simulink library "Susp_AxleTA2PRNoSteer"  (R2023b)
settings: Solver=ode23t  StartTime=0.0  StopTime=10.0  RelTol=1e-3
undefined symbols (not defined in the file): Axle1D, AxleIn, Init, RaceFix, RaceSpin, Susp, Visual, X, Y, Z
libraries: sm_lib x46, Suspension_Utilities x10, Susp_Components x5, Linkage_Shock x2, Susp_AxleTA4Watts x2, Linkage_Spring x2, Linkage_Bumpstop x1, Susp_TwistBeam x1
(part 1 of 2)
Description:
  | Component of Simscape Vehicle Templates Library
  | 
  | Copyright 2018-2025 The MathWorks, Inc.
settings Model: Creator=mwalker  LastModifiedBy=smiller
settings SolverCC: AlgebraicLoopSolver=TrustRegion
settings DataIOCC: ReturnWorkspaceOutputs=off
settings DebuggingCC: UnconnectedInputMsg=warning  UnconnectedOutputMsg=warning  UnconnectedLineMsg=warning  ArithmeticOperatorsInVariantConditions=warning
settings ModelReferenceCC: EnableRefExpFcnMdlSchedulingChecks=on
settings SFSimCC: CustomCodeUndefinedFunction=UseInterfaceOnly

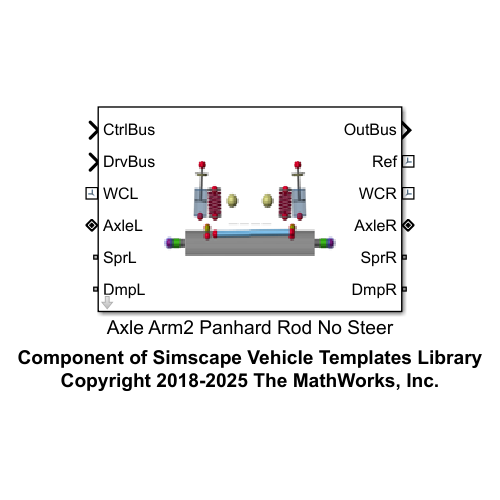
[thumbnail: Simulink's stored preview of the top-level diagram]
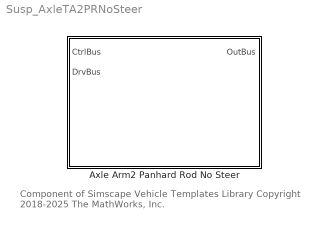
== system Susp_AxleTA2PRNoSteer ==
  note: Component of Simscape Vehicle Templates Library
      | Copyright 2018-2025 The MathWorks, Inc.
  Axle Arm2 Panhard Rod No Steer : Subsystem  VariantControl=LiveAxle  mask(Rigid Axle 2 Trailing Arm Panhard Rod Suspension, No Steer){Init=Init, hp_damper_topL=Susp.AxleTA2PR.Damper.sTopL.Value, hp_damper_topR=Susp.AxleTA2PR.Damper.sTopR.Value, hp_damper_botL=Susp.AxleTA2PR.Damper.sBottomL.Value, hp_damper_botR=Susp.AxleTA2PR.Damper.sBottomR.Value, hp_spring_topL=Susp.AxleTA2PR.Spring.sTopL.Value, hp_spring_topR=Susp.AxleTA2PR.Spring.sTopR.Value, hp_spring_botL=Susp.AxleTA2PR.Spring.sBottomL.Value, hp_spring_botR=Susp.AxleTA2PR.Spring.sBottomR.Value, hp_arm_body=Susp.AxleTA2PR.TrailingArm.sBody.Value, hp_arm_axleL=Susp.AxleTA2PR.TrailingArm.sAxleL.Value, hp_arm_axleR=Susp.AxleTA2PR.TrailingArm.sAxleR.Value, hp_pan_body=Susp.AxleTA2PR.PanhardRod.sBody.Value, hp_pan_axle=Susp.AxleTA2PR.PanhardRod.sAxle.Value, hp_axle_cg=Susp.AxleTA2PR.Axle.sCG.Value, hp_whl_ctrL=Susp.AxleTA2PR.Axle.sWheelCentreL.Value, hp_whl_ctrR=Susp.AxleTA2PR.Axle.sWheelCentreR.Value, hp_axle_outboardL=Susp.AxleTA2PR.Axle.sOutboardL.Value, hp_axle_outboardR=Susp.AxleTA2PR.Axle.sOutboardR.Value, hp_bumpstop_body=Susp.AxleTA2PR.Bumpstop.sBody.Value, hp_bumpstop_axle=Susp.AxleTA2PR.Bumpstop.sAxle.Value, axle_mass=Susp.AxleTA2PR.Axle.m.Value, axle_k=Susp.AxleTA2PR.Axle.k.Value, axle_d=Susp.AxleTA2PR.Axle.d.Value, stub_axle_len=Susp.AxleTA2PR.StubAxle.xAxle.Value, stub_axle_mass=Susp.AxleTA2PR.StubAxle.m.Value, axle_whlc_to_bearing=Susp.AxleTA2PR.Axle.xWCtoBearing.Value, arm_mass=Susp.AxleTA2PR.TrailingArm.m.Value, panhard_mass=Susp.AxleTA2PR.PanhardRod.m.Value, Arm_to_Body=Susp.AxleTA2PR.Arm_to_Body, Rod_to_Body=Susp.AxleTA2PR.Rod_to_Body, Rod_to_Axle=Susp.AxleTA2PR.Rod_to_Axle, DamperL_to_Body=Susp.AxleTA2PR.DamperL_to_Body, DamperR_to_Body=Susp.AxleTA2PR.DamperR_to_Body, DamperL_to_Axle=Susp.AxleTA2PR.DamperL_to_Axle, DamperR_to_Axle=Susp.AxleTA2PR.DamperR_to_Axle, clr_arm=Visual.UpperArm.clr, opc_arm=Visual.part.opc, radius_arm=Visual.UpperArm.rad, clr_rod=Visual.Pushrod.clr, opc_rod=Visual.part.opc, radius_rod=Visual.Pushrod.rad, clr_conn_links=Visual.hp.clr, opc_conn_links=Visual.hp.opc, size_conn_links=Visual.hp.rad, clr_stub_axle=Visual.Axle.clr, opc_stub_axle=Visual.part.opc, rad_stub_axle=Visual.Axle.rad, piston_mass=Susp.AxleTA2PR.Shock.mPiston.Value, cyl_mass=Susp.AxleTA2PR.Shock.mCylinder.Value, shock_xmax=Susp.AxleTA2PR.Endstop.xMax.Value, shock_xmin=Susp.AxleTA2PR.Endstop.xMin.Value, spring_mass=Susp.AxleTA2PR.Spring.m.Value, Bumpstop_Type=Susp.AxleTA2PR.Bumpstop.class.Value, bumpstop_height=Susp.AxleTA2PR.Bumpstop.xHeight.Value, bumpstop_k=Susp.AxleTA2PR.Bumpstop.K.Value, bumpstop_d=Susp.AxleTA2PR.Bumpstop.d.Value, bumpstop_xTrans=Susp.AxleTA2PR.Bumpstop.xTransition.Value, bumpstop_ptcld=Susp.AxleTA2PR.Bumpstop.sPointCloud.Value, Beam=Susp.AxleTA2PR.Beam, Beam_Flexibility=Susp.AxleTA2PR.Beam.class.Value}
      mask prompts: Init "Initial Wheel Speed (rad/s)"; hp_damper_topL "HP Damper Top, Left [xyz] (m)"; hp_damper_topR "HP Damper Top, Right [xyz] (m)"; hp_damper_botL "HP Damper Bottom, Left [xyz] (m)"; hp_damper_botR "HP Damper Bottom, Right [xyz] (m)"; hp_spring_topL "HP Spring Top, Left [xyz] (m)"; hp_spring_topR "HP Spring Top, Right [xyz] (m)"; hp_spring_botL "HP Spring Bottom, Left [xyz] (m)"; hp_spring_botR "HP Spring Bottom, Right [xyz] (m)"; hp_arm_body "HP Trailing Arm to Body [xyz] (m)"; hp_arm_axleL "HP Trailing Arm to Axle, Left [xyz] (m)"; hp_arm_axleR "HP Trailing Arm to Axle, Right [xyz] (m)"; hp_pan_body "HP Panhard Rod to Body [xyz] (m)"; hp_pan_axle "HP Panhard Rod to Axle [xyz] (m)"; hp_axle_cg "HP Axle CG [xyz] (m)"; hp_whl_ctrL "HP Wheel Center, Left [xyz] (m)"; hp_whl_ctrR "HP Wheel Center, Right [xyz] (m)"; hp_axle_outboardL "HP Axle Outboard, Left [xyz] (m)"; hp_axle_outboardR "HP Axle Outboard, Right [xyz] (m)"; hp_bumpstop_body "HP Bumpstop Body [xyz] (m)"; hp_bumpstop_axle "HP Bumpstop Axle [xyz] (m)"; axle_mass "Axle Mass (kg)"; axle_k "Axle Stiffness (N*m/deg)"; axle_d "Axle Damping (N*m/(deg/s))"; stub_axle_len "Stub Axle Length (m)"; stub_axle_mass "Stub Axle Mass (kg)"; axle_whlc_to_bearing "Distance Wheel Ctr to Bearing (m)"; arm_mass "Trailing Arm Mass (kg)"; panhard_mass "Panhard Rod (kg)"; Arm_to_Body "Arm Body Connection"; Rod_to_Body "Rod Body Connection"; Rod_to_Axle "Rod Axle Connection"; DamperL_to_Body "Damper Left Body Connection"; DamperR_to_Body "Damper Right Body Connection"; DamperL_to_Axle "Damper Left Axle Connection"; DamperR_to_Axle "Damper Right Axle Connection"; clr_arm "Arm Color [R G B]"; opc_arm "Arm Opacity"; radius_arm "Arm Radius (m)"; clr_rod "Rod Color [R G B]"; opc_rod "Rod Opacity"; radius_rod "Rod Radius (m)"; clr_conn_links "Connection Color [R G B]"; opc_conn_links "Connection Opacity"; size_conn_links "Connection Radius (m)"; clr_stub_axle "Stub Axle [R G B]"; opc_stub_axle "Stub Axle Opacity"; rad_stub_axle "Stub Axle Radius (m)"; piston_mass "Piston Mass (kg)"; cyl_mass "Cylinder Mass (kg)"; shock_xmax "Upper Limit Bumpstop (m)"; shock_xmin "Lower Limit Bumpstop (m)"; spring_mass "Spring Mass (kg)"; Bumpstop_Type "Type"; bumpstop_height "Height (m)"; bumpstop_k "Stiffness (N/m)"; bumpstop_d "Damping (N/(m/s))"; bumpstop_xTrans "Transition Depth (m)"; bumpstop_ptcld "Point Cloud [xyz] (m)"; Beam "Beam Parameters"; Beam_Flexibility "Beam Flexibility"
      mask help: Models a rigid axle connecting two wheel with two trailing arms and a panhard rod. The wheels are not steerable.
      mask init:
      | bh = gcb;
      | set_param([bh '/Axle'],'popup_axle_flex',Beam_Flexibility);
      mask DialogControl cont_hp Prompt: Hardpoints, Axes
      mask DialogControl cont_parts Prompt: Parts
      mask DialogControl Container7 Prompt: Visualization
      mask DialogControl cont_shock Prompt: Shock
      mask DialogControl cont_bumpstop Prompt: Bumpstop
      mask DialogControl cont_beam Prompt: Beam
      mask Display: image('sm_car_vehicle_susp_axleta2prnst_IMAGE.png');

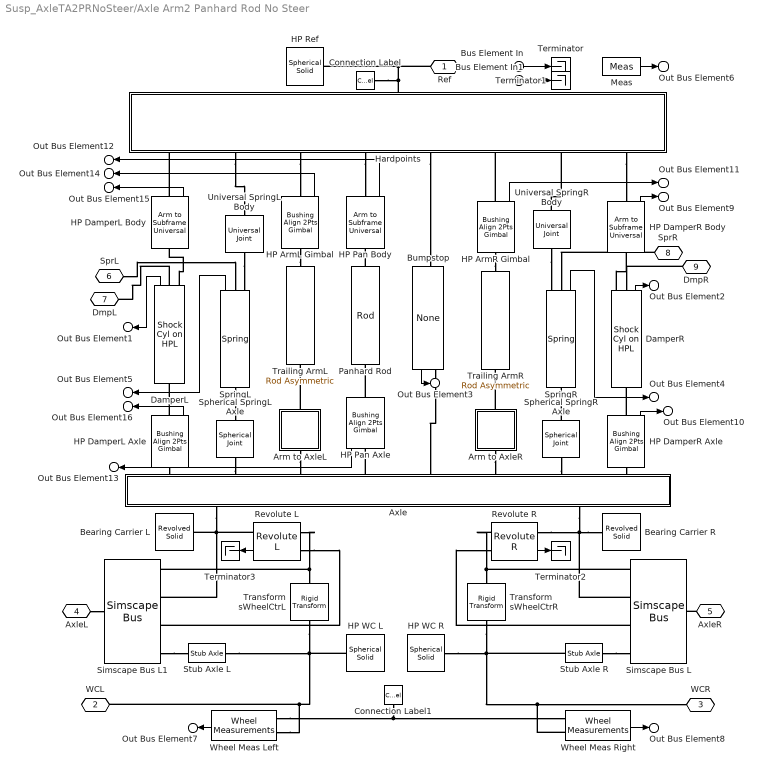
== system Susp_AxleTA2PRNoSteer/Axle Arm2 Panhard Rod No Steer ==
  Bus Element In1 : Inport  PortName=CtrlBus
  Bus Element In : Inport  Port=2  PortName=DrvBus
  Arm to AxleL : Subsystem  VariantControl=Kinematic
  Arm to AxleR : Subsystem  VariantControl=Kinematic
  Axle : Subsystem  mask{hp_axle_outboardL=hp_axle_outboardL, hp_axle_outboardR=hp_axle_outboardR, popup_axle_flex=Beam, beam_rho=Beam.density.Value, xc_x=Beam.xcX.Value, xc_z=Beam.xcZ.Value, beam_E=Beam.E.Value, beam_nu=Beam.nu.Value, beam_zeta=Beam.zDamping.Value, beam_numElements=Beam.numElements.Value, clr_beam=Visual.clr.orangedark, opc_beam=Visual.part.opc}
      mask prompts: hp_axle_outboardL "Axle Outboard Left [x y z] (m)"; hp_axle_outboardR "Axle Outboard Right [x y z] (m)"; popup_axle_flex "Flexibility"; beam_rho "Beam Density (kg/m^3)"; xc_x "Extrusion Points X (m)"; xc_z "Extrusion Points Z (m)"; beam_E "Young's Modulus (GPa)"; beam_nu "Poisson's Ratio"; beam_zeta "Damping Constant (sec)"; beam_numElements "Number of Beam Elements"; clr_beam "Beam Color [RGB]"; opc_beam "Beam Opacity (0-1)"
      mask init:
      | bh = gcb;
      | set_param([bh '/Axle'],'LabelModeActiveChoice',get_param(bh,'popup_axle_flex'));
      mask TypeOptions popup_axle_flex: Torsional | Beam
      mask DialogControl cont_axle_flex Prompt: Axle Flex
      mask DialogControl cont_vis Prompt: Visualization
  Bearing Carrier L : sm_lib/Body Elements/Revolved Solid  GraphicAmbientColor=[0.15 0.15 0.15 1.0]  BasedOnType=Density  CenterOfMass=[0 0 0]  CenterOfMassUnits=m  GraphicDiffuseColor=Visual.Upright.clr  ExportConvexHullGeometry=off  Density=1000  DensityUnits=kg/m^3  DoExposeReferenceFrame=on  GraphicEmissiveColor=[0.0 0.0 0.0 1.0]  ExportEntireGeometry=off  SerializedFrames=<Frames/>  MarkerShape=Sphere  MarkerSize=10  GraphicType=FromGeometry  InertiaType=CalculateFromGeometry  Mass=1  MassUnits=kg  MomentsOfInertia=[1 1 1]  MomentsOfInertiaUnits=kg*m^2  GraphicOpacity=0.5  ProductsOfInertia=[0 0 0]  ProductsOfInertiaUnits=kg*m^2  RevolutionCrossSection=[1.2 0.5; 1.1 0.5; 1.1 -0.5; 1.2 -0.5].*[rad_stub_axle 0.05]  RevolutionCrossSectionUnits=m  RevolutionAngle=180  RevolutionAngleUnits=deg  RevolutionExtent=Full  GraphicShininess=75  GraphicSpecularColor=[0.5 0.5 0.5 1.0]  GraphicVisPropType=SimpleVisualProperties
  Bearing Carrier R : sm_lib/Body Elements/Revolved Solid  GraphicAmbientColor=[0.15 0.15 0.15 1.0]  BasedOnType=Density  CenterOfMass=[0 0 0]  CenterOfMassUnits=m  GraphicDiffuseColor=Visual.Upright.clr  ExportConvexHullGeometry=off  Density=1000  DensityUnits=kg/m^3  DoExposeReferenceFrame=on  GraphicEmissiveColor=[0.0 0.0 0.0 1.0]  ExportEntireGeometry=off  SerializedFrames=<Frames/>  MarkerShape=Sphere  MarkerSize=10  GraphicType=FromGeometry  InertiaType=CalculateFromGeometry  Mass=1  MassUnits=kg  MomentsOfInertia=[1 1 1]  MomentsOfInertiaUnits=kg*m^2  GraphicOpacity=0.5  ProductsOfInertia=[0 0 0]  ProductsOfInertiaUnits=kg*m^2  RevolutionCrossSection=[1.2 0.5; 1.1 0.5; 1.1 -0.5; 1.2 -0.5].*[rad_stub_axle 0.05]  RevolutionCrossSectionUnits=m  RevolutionAngle=180  RevolutionAngleUnits=deg  RevolutionExtent=Full  GraphicShininess=75  GraphicSpecularColor=[0.5 0.5 0.5 1.0]  GraphicVisPropType=SimpleVisualProperties
  Bumpstop : Linkage_Bumpstop/None  VariantControl=Choice  LabelModeActiveChoice=SphereSurface  VariantLabel=Bumpstop_Type
  Connection Label : ConnectionLabel  Label=Ref
  Connection Label1 : ConnectionLabel  Label=Ref
  DamperL : Linkage_Shock/Shock Cyl on HPL  VariantControl=CylDownCylBot  shock_pist_mass=piston_mass  shock_cyl_mass=cyl_mass  hp_spr_top=hp_damper_topL  hp_spr_bot=hp_damper_botL  up_lim_bumpstop=shock_xmax  low_lim_bumpstop=shock_xmin  clr_conn_shock=Visual.hp.clr  opc_conn_shock=Visual.hp.opc  size_conn_shock=Visual.hp.rad  clr_shock_cyl=Visual.clr.blue  opc_shock_cyl=Visual.part.opc  radius_shock_cyl=0.05  clr_shock_piston=Visual.clr.gray  opc_shock_piston=Visual.part.opc  clr_shock_bumpstop=Visual.clr.yellowpale  opc_shock_bumpstop=Visual.part.opc  deadvol_len_shock_cyl=Visual.Shock.dead_length  piston_len_shock=Visual.Shock.piston.len  cyl_cap_len_shock=Visual.Shock.cap.len  bumpstop_len_shock=Visual.Shock.bumpstop.len
  DamperR : Linkage_Shock/Shock Cyl on HPL  VariantControl=CylDownCylBot  shock_pist_mass=piston_mass  shock_cyl_mass=cyl_mass  hp_spr_top=hp_damper_topR  hp_spr_bot=hp_damper_botR  up_lim_bumpstop=shock_xmax  low_lim_bumpstop=shock_xmin  clr_conn_shock=Visual.hp.clr  opc_conn_shock=Visual.hp.opc  size_conn_shock=Visual.hp.rad  clr_shock_cyl=Visual.clr.blue  opc_shock_cyl=Visual.part.opc  radius_shock_cyl=0.05  clr_shock_piston=Visual.clr.gray  opc_shock_piston=Visual.part.opc  clr_shock_bumpstop=Visual.clr.yellowpale  opc_shock_bumpstop=Visual.part.opc  deadvol_len_shock_cyl=Visual.Shock.dead_length  piston_len_shock=Visual.Shock.piston.len  cyl_cap_len_shock=Visual.Shock.cap.len  bumpstop_len_shock=Visual.Shock.bumpstop.len
  HP DamperL Axle : Suspension_Utilities/Bushing Align 2Pts Gimbal  VariantControl=Variant1  LabelModeActiveChoice=Bushing_Tr3Ro3  popup_leftRight=Left  hp_joint=hp_damper_botL  Connection=DamperL_to_Axle  VariantLabel=DamperL_to_Axle.class.Value  checkbox_setTargets=off
  HP DamperL Body : Suspension_Utilities/Arm to Subframe Universal  VariantControl=Variant1  LabelModeActiveChoice=Bushing_AxRad  popup_leftRight=Left  hp_joint=hp_damper_topL  Connection=DamperL_to_Body  VariantLabel=DamperL_to_Body.class.Value  checkbox_setTargets=off
      settings: AttributesFormatString=%<ActiveVariant>
  HP DamperR Axle : Suspension_Utilities/Bushing Align 2Pts Gimbal  VariantControl=Variant1  LabelModeActiveChoice=Bushing_Tr3Ro3  popup_leftRight=Left  hp_joint=hp_damper_botR  Connection=DamperR_to_Axle  VariantLabel=DamperR_to_Axle.class.Value  checkbox_setTargets=off
  HP DamperR Body : Suspension_Utilities/Arm to Subframe Universal  VariantControl=Variant1  LabelModeActiveChoice=Bushing_AxRad  popup_leftRight=Left  hp_joint=hp_damper_topR  Connection=DamperR_to_Body  VariantLabel=DamperR_to_Body.class.Value  checkbox_setTargets=off
      settings: AttributesFormatString=%<ActiveVariant>
  HP Pan Axle : Suspension_Utilities/Bushing Align 2Pts Gimbal  VariantControl=Variant1  LabelModeActiveChoice=Bushing_Tr3Ro3  popup_leftRight=Left  hp_joint=hp_pan_axle  Connection=Rod_to_Axle  VariantLabel=Rod_to_Axle.class.Value  checkbox_setTargets=off
      settings: AttributesFormatString=%<ActiveVariant>
  HP Pan Body : Suspension_Utilities/Arm to Subframe Universal  VariantControl=Variant1  LabelModeActiveChoice=Bushing_AxRad  popup_leftRight=Left  hp_joint=hp_pan_body  Connection=Rod_to_Body  VariantLabel=Rod_to_Body.class.Value  checkbox_setTargets=off
      settings: AttributesFormatString=%<ActiveVariant>
  HP ArmL Gimbal : Suspension_Utilities/Bushing Align 2Pts Gimbal  VariantControl=Variant1  LabelModeActiveChoice=Bushing_Tr3Ro3  popup_leftRight=Left  hp_joint=hp_arm_body  Connection=Arm_to_Body  VariantLabel=Arm_to_Body.class.Value  checkbox_setTargets=on
  HP ArmR Gimbal : Suspension_Utilities/Bushing Align 2Pts Gimbal  VariantControl=Variant1  LabelModeActiveChoice=Bushing_Tr3Ro3  popup_leftRight=Left  hp_joint=hp_arm_body  Connection=Arm_to_Body  VariantLabel=Arm_to_Body.class.Value  checkbox_setTargets=on
  HP Ref : sm_lib/Body Elements/Spherical Solid  GraphicAmbientColor=[0.15 0.15 0.15 1.0]  BasedOnType=Density  CenterOfMass=[0 0 0]  CenterOfMassUnits=m  GraphicDiffuseColor=Visual.hp.clr  Density=1000  DensityUnits=kg/m^3  DoExposeReferenceFrame=on  GraphicEmissiveColor=[0.0 0.0 0.0 1.0]  ExportEntireGeometry=off  SerializedExposedGeometries=<ExposedGeometries/>  SerializedFrames=<Frames/>  MarkerShape=Sphere  MarkerSize=10  GraphicType=FromGeometry  InertiaType=CalculateFromGeometry  Mass=1  MassUnits=kg  MomentsOfInertia=[1 1 1]  MomentsOfInertiaUnits=kg*m^2  GraphicOpacity=Visual.hp.opc  ProductsOfInertia=[0 0 0]  ProductsOfInertiaUnits=kg*m^2  GraphicShininess=75  GraphicSpecularColor=[0.5 0.5 0.5 1.0]  SphereRadius=Visual.hp.rad  SphereRadiusUnits=m  GraphicVisPropType=SimpleVisualProperties
  HP WC L : sm_lib/Body Elements/Spherical Solid  GraphicAmbientColor=[0.15 0.15 0.15 1.0]  BasedOnType=Density  CenterOfMass=[0 0 0]  CenterOfMassUnits=m  GraphicDiffuseColor=Visual.hp.clr  Density=1000  DensityUnits=kg/m^3  DoExposeReferenceFrame=on  GraphicEmissiveColor=[0.0 0.0 0.0 1.0]  ExportEntireGeometry=off  SerializedExposedGeometries=<ExposedGeometries/>  SerializedFrames=<Frames/>  MarkerShape=Sphere  MarkerSize=10  GraphicType=FromGeometry  InertiaType=CalculateFromGeometry  Mass=1  MassUnits=kg  MomentsOfInertia=[1 1 1]  MomentsOfInertiaUnits=kg*m^2  GraphicOpacity=Visual.hp.opc  ProductsOfInertia=[0 0 0]  ProductsOfInertiaUnits=kg*m^2  GraphicShininess=75  GraphicSpecularColor=[0.5 0.5 0.5 1.0]  SphereRadius=Visual.hp.rad  SphereRadiusUnits=m  GraphicVisPropType=SimpleVisualProperties
  HP WC R : sm_lib/Body Elements/Spherical Solid  GraphicAmbientColor=[0.15 0.15 0.15 1.0]  BasedOnType=Density  CenterOfMass=[0 0 0]  CenterOfMassUnits=m  GraphicDiffuseColor=Visual.hp.clr  Density=1000  DensityUnits=kg/m^3  DoExposeReferenceFrame=on  GraphicEmissiveColor=[0.0 0.0 0.0 1.0]  ExportEntireGeometry=off  SerializedExposedGeometries=<ExposedGeometries/>  SerializedFrames=<Frames/>  MarkerShape=Sphere  MarkerSize=10  GraphicType=FromGeometry  InertiaType=CalculateFromGeometry  Mass=1  MassUnits=kg  MomentsOfInertia=[1 1 1]  MomentsOfInertiaUnits=kg*m^2  GraphicOpacity=Visual.hp.opc  ProductsOfInertia=[0 0 0]  ProductsOfInertiaUnits=kg*m^2  GraphicShininess=75  GraphicSpecularColor=[0.5 0.5 0.5 1.0]  SphereRadius=Visual.hp.rad  SphereRadiusUnits=m  GraphicVisPropType=SimpleVisualProperties
  Hardpoints : Subsystem
  Meas : Susp_TwistBeam/TwistBeam/Meas  SystemSampleTime=-1  VariantActivationTime=update diagram  AllowFlexibleInterface=on  Latency=0  AutoFrameSizeCalculation=off
  Panhard Rod : Susp_Components/Rod  VariantControl=Steer  popup_leftRight=Left  hp_in=hp_pan_body  hp_out=hp_pan_axle  rod_mass=panhard_mass  clr_conn_rod=clr_conn_links  opc_conn_rod=opc_conn_links  size_conn_rod=size_conn_links  clr_rod=clr_rod  opc_rod=opc_rod  radius_rod=radius_rod
  Revolute L : Susp_AxleTA4Watts/Axle Arm4 Watts Link/Revolute L  whl_spd_init_l=Init.nWheel.Value(1)
  Revolute R : Susp_AxleTA4Watts/Axle Arm4 Watts Link/Revolute R  whl_spd_init_r=Init.nWheel.Value(2)
  Simscape Bus L : SimscapeBus  HierarchyStrings=RaceSpin;RaceFix;Axle1D;AxleIn
  Simscape Bus L1 : SimscapeBus  HierarchyStrings=RaceSpin;RaceFix;Axle1D;AxleIn
  Spherical SpringL Axle : sm_lib/Joints/Spherical Joint  JointMode=Normal  SenseConstraintForce=off  SenseConstraintForceX=off  SenseConstraintForceY=off  SenseConstraintForceZ=off  SenseConstraintTorque=off  SenseConstraintTorqueX=off  SenseConstraintTorqueY=off  SenseConstraintTorqueZ=off  SenseTotalForce=off  SenseTotalForceX=off  SenseTotalForceY=off  SenseTotalForceZ=off  SenseTotalTorque=off  SenseTotalTorqueX=off  SenseTotalTorqueY=off  SenseTotalTorqueZ=off  CompositeWrenchDir=FollowerOnBase  CompositeWrenchFrame=BaseFrame  EqPosRotationMethod=None  EqPosRotationAngleUnits=deg  EqPosRotationStandardAxis=+Z  EqPosRotationAngle=0.0  EqPosRotationArbitraryAxis=[0 0 1]  EqPosFollAlignAxisA=+X  EqPosBaseAlignAxisA=+Y  EqPosFollAlignAxisB=+Y  EqPosBaseAlignAxisB=+Z  EqPosRotationSequenceAxes=FollowerAxes  EqPosRotationSequence=XYX  EqPosRotationSequenceAngles=[0 0 0]  EqPosRotationSequenceAnglesUnits=deg  EqPosRotationMatrix=[1 0 0; 0 1 0; 0 0 1]  EqPosQuaternion=[1 0 0 0]  SpringStiffness=0  SpringStiffnessUnits=N*m/deg  DampingCoefficient=0  DampingCoefficientUnits=N*m/(deg/s)  ActuateTorqueX=off  ActuateTorqueY=off  ActuateTorqueZ=off  ActuateTorque=off  TorqueActuationMode=NoTorque  MotionActuationMode=ComputedMotion  ActuationFrame=BaseFrame  SensePosition=off  SenseVelocityX=off  SenseVelocityY=off  SenseVelocityZ=off  SenseVelocity=off  SenseAccelerationX=off  SenseAccelerationY=off  SenseAccelerationZ=off  SenseAcceleration=off  SenseTorqueX=off  SenseTorqueY=off  SenseTorqueZ=off  SenseTorqueForce=off  SenseLowerLimitTorqueMag=off  SenseUpperLimitTorqueMag=off  SensingFrame=BaseFrame  LowerLimitSpecify=off  LowerLimitBound=15  LowerLimitBoundUnits=deg  LowerLimitStiffness=1e4  LowerLimitStiffnessUnits=N*m/deg  LowerLimitDamping=10  LowerLimitDampingUnits=N*m/(deg/s)  LowerLimitTransitionRegionWidth=0.1  LowerLimitTransitionRegionWidthUnits=deg  UpperLimitSpecify=off  UpperLimitBound=45  UpperLimitBoundUnits=deg  UpperLimitStiffness=1e4  UpperLimitStiffnessUnits=N*m/deg  UpperLimitDamping=10  UpperLimitDampingUnits=N*m/(deg/s)  UpperLimitTransitionRegionWidth=0.1  UpperLimitTransitionRegionWidthUnits=deg  PositionTargetRotationMethod=None  PositionTargetRotationAngleUnits=deg  PositionTargetRotationStandardAxis=+Z  PositionTargetRotationAngle=0.0  PositionTargetRotationArbitraryAxis=[0 0 1]  PositionTargetFollAlignAxisA=+X  PositionTargetBaseAlignAxisA=+Y  PositionTargetFollAlignAxisB=+Y  PositionTargetBaseAlignAxisB=+Z  PositionTargetRotationSequenceAxes=FollowerAxes  PositionTargetRotationSequence=XYX  PositionTargetRotationSequenceAngles=[0 0 0]  PositionTargetRotationSequenceAnglesUnits=deg  PositionTargetRotationMatrix=[1 0 0; 0 1 0; 0 0 1]  PositionTargetQuaternion=[1 0 0 0]  PositionTargetSpecify=off  PositionTargetPriority=High  VelocityTargetValue=[0 0 0]  VelocityTargetValueUnits=deg/s  VelocityTargetSpecify=off  VelocityTargetPriority=High  VelocityTargetInFollowerFrame=on
  Spherical SpringR Axle : sm_lib/Joints/Spherical Joint  JointMode=Normal  SenseConstraintForce=off  SenseConstraintForceX=off  SenseConstraintForceY=off  SenseConstraintForceZ=off  SenseConstraintTorque=off  SenseConstraintTorqueX=off  SenseConstraintTorqueY=off  SenseConstraintTorqueZ=off  SenseTotalForce=off  SenseTotalForceX=off  SenseTotalForceY=off  SenseTotalForceZ=off  SenseTotalTorque=off  SenseTotalTorqueX=off  SenseTotalTorqueY=off  SenseTotalTorqueZ=off  CompositeWrenchDir=FollowerOnBase  CompositeWrenchFrame=BaseFrame  EqPosRotationMethod=None  EqPosRotationAngleUnits=deg  EqPosRotationStandardAxis=+Z  EqPosRotationAngle=0.0  EqPosRotationArbitraryAxis=[0 0 1]  EqPosFollAlignAxisA=+X  EqPosBaseAlignAxisA=+Y  EqPosFollAlignAxisB=+Y  EqPosBaseAlignAxisB=+Z  EqPosRotationSequenceAxes=FollowerAxes  EqPosRotationSequence=XYX  EqPosRotationSequenceAngles=[0 0 0]  EqPosRotationSequenceAnglesUnits=deg  EqPosRotationMatrix=[1 0 0; 0 1 0; 0 0 1]  EqPosQuaternion=[1 0 0 0]  SpringStiffness=0  SpringStiffnessUnits=N*m/deg  DampingCoefficient=0  DampingCoefficientUnits=N*m/(deg/s)  ActuateTorqueX=off  ActuateTorqueY=off  ActuateTorqueZ=off  ActuateTorque=off  TorqueActuationMode=NoTorque  MotionActuationMode=ComputedMotion  ActuationFrame=BaseFrame  SensePosition=off  SenseVelocityX=off  SenseVelocityY=off  SenseVelocityZ=off  SenseVelocity=off  SenseAccelerationX=off  SenseAccelerationY=off  SenseAccelerationZ=off  SenseAcceleration=off  SenseTorqueX=off  SenseTorqueY=off  SenseTorqueZ=off  SenseTorqueForce=off  SenseLowerLimitTorqueMag=off  SenseUpperLimitTorqueMag=off  SensingFrame=BaseFrame  LowerLimitSpecify=off  LowerLimitBound=15  LowerLimitBoundUnits=deg  LowerLimitStiffness=1e4  LowerLimitStiffnessUnits=N*m/deg  LowerLimitDamping=10  LowerLimitDampingUnits=N*m/(deg/s)  LowerLimitTransitionRegionWidth=0.1  LowerLimitTransitionRegionWidthUnits=deg  UpperLimitSpecify=off  UpperLimitBound=45  UpperLimitBoundUnits=deg  UpperLimitStiffness=1e4  UpperLimitStiffnessUnits=N*m/deg  UpperLimitDamping=10  UpperLimitDampingUnits=N*m/(deg/s)  UpperLimitTransitionRegionWidth=0.1  UpperLimitTransitionRegionWidthUnits=deg  PositionTargetRotationMethod=None  PositionTargetRotationAngleUnits=deg  PositionTargetRotationStandardAxis=+Z  PositionTargetRotationAngle=0.0  PositionTargetRotationArbitraryAxis=[0 0 1]  PositionTargetFollAlignAxisA=+X  PositionTargetBaseAlignAxisA=+Y  PositionTargetFollAlignAxisB=+Y  PositionTargetBaseAlignAxisB=+Z  PositionTargetRotationSequenceAxes=FollowerAxes  PositionTargetRotationSequence=XYX  PositionTargetRotationSequenceAngles=[0 0 0]  PositionTargetRotationSequenceAnglesUnits=deg  PositionTargetRotationMatrix=[1 0 0; 0 1 0; 0 0 1]  PositionTargetQuaternion=[1 0 0 0]  PositionTargetSpecify=off  PositionTargetPriority=High  VelocityTargetValue=[0 0 0]  VelocityTargetValueUnits=deg/s  VelocityTargetSpecify=off  VelocityTargetPriority=High  VelocityTargetInFollowerFrame=on
  SpringL : Linkage_Spring/Spring  spring_mass=spring_mass  hp_spr_top=hp_spring_topL  hp_spr_bot=hp_spring_botL  clr_conn_shock=Visual.hp.clr  opc_conn_shock=Visual.hp.opc  size_conn_shock=Visual.hp.rad  clr_spring_cyl=Visual.Spring.cyl.clr  opc_shock_cyl=Visual.Spring.cyl.opc  radius_shock_cyl=Visual.Spring.cyl.rad  clr_spring_cap=Visual.Spring.cap.clr  opc_spring_cap=Visual.part.opc  clr_spring_coil=Visual.Spring.coil.clr  opc_spring_coil=Visual.Spring.coil.opc  cyl_cap_len_shock=Visual.Spring.cap.len
  SpringR : Linkage_Spring/Spring  spring_mass=spring_mass  hp_spr_top=hp_spring_topR  hp_spr_bot=hp_spring_botR  clr_conn_shock=Visual.hp.clr  opc_conn_shock=Visual.hp.opc  size_conn_shock=Visual.hp.rad  clr_spring_cyl=Visual.Spring.cyl.clr  opc_shock_cyl=Visual.Spring.cyl.opc  radius_shock_cyl=Visual.Spring.cyl.rad  clr_spring_cap=Visual.Spring.cap.clr  opc_spring_cap=Visual.part.opc  clr_spring_coil=Visual.Spring.coil.clr  opc_spring_coil=Visual.Spring.coil.opc  cyl_cap_len_shock=Visual.Spring.cap.len
  Stub Axle L : Susp_Components/Stub Axle  popup_leftRight=Left  stub_axle_len=stub_axle_len  stub_axle_mass=stub_axle_mass  clr_stub_axle=clr_stub_axle  opc_stub_axle=opc_stub_axle  rad_stub_axle=rad_stub_axle
  Stub Axle R : Susp_Components/Stub Axle  popup_leftRight=Right  stub_axle_len=stub_axle_len  stub_axle_mass=stub_axle_mass  clr_stub_axle=clr_stub_axle  opc_stub_axle=opc_stub_axle  rad_stub_axle=rad_stub_axle
  Terminator{,1..3} (4 alike) : Terminator
  Trailing ArmL : Susp_Components/Rod Asymmetric  VariantControl=Steer  hp_in=hp_arm_body  hp_out=hp_arm_axleL  rod_mass=arm_mass  clr_conn_rod=clr_conn_links  opc_conn_rod=opc_conn_links  size_conn_rod=size_conn_links  clr_rod=clr_arm  opc_rod=opc_arm  radius_rod=radius_arm
  Trailing ArmR : Susp_Components/Rod Asymmetric  VariantControl=Steer  hp_in=hp_arm_body.*[1 -1 1]  hp_out=hp_arm_axleR  rod_mass=arm_mass  clr_conn_rod=clr_conn_links  opc_conn_rod=opc_conn_links  size_conn_rod=size_conn_links  clr_rod=clr_arm  opc_rod=opc_arm  radius_rod=radius_arm
  Transform sWheelCtrL : sm_lib/Frames and Transforms/Rigid Transform  TranslationMethod=StandardAxis  TranslationStandardOffset=axle_whlc_to_bearing  TranslationStandardOffsetUnits=m  TranslationStandardAxis=-Z  TranslationCartesianOffset=[0 0 0]  TranslationCartesianOffsetUnits=m  TranslationROffset=0  TranslationROffsetUnits=m  TranslationZOffset=0  TranslationZOffsetUnits=m  TranslationThetaOffset=0  TranslationThetaOffsetUnits=deg  RotationMethod=None  RotationAngleUnits=deg  RotationStandardAxis=+X  RotationAngle=-90  RotationArbitraryAxis=[0 0 1]  FollAlignAxisA=+X  BaseAlignAxisA=+Y  FollAlignAxisB=+Y  BaseAlignAxisB=+Z  RotationSequenceAxes=FollowerAxes  RotationSequence=XYX  RotationSequenceAngles=[0 0 0]  RotationSequenceAnglesUnits=deg  RotationMatrix=[1 0 0; 0 1 0; 0 0 1]  Quaternion=[1 0 0 0]
  Transform sWheelCtrR : sm_lib/Frames and Transforms/Rigid Transform  TranslationMethod=StandardAxis  TranslationStandardOffset=axle_whlc_to_bearing  TranslationStandardOffsetUnits=m  TranslationStandardAxis=+Z  TranslationCartesianOffset=[0 0 0]  TranslationCartesianOffsetUnits=m  TranslationROffset=0  TranslationROffsetUnits=m  TranslationZOffset=0  TranslationZOffsetUnits=m  TranslationThetaOffset=0  TranslationThetaOffsetUnits=deg  RotationMethod=None  RotationAngleUnits=deg  RotationStandardAxis=+X  RotationAngle=-90  RotationArbitraryAxis=[0 0 1]  FollAlignAxisA=+X  BaseAlignAxisA=+Y  FollAlignAxisB=+Y  BaseAlignAxisB=+Z  RotationSequenceAxes=FollowerAxes  RotationSequence=XYX  RotationSequenceAngles=[0 0 0]  RotationSequenceAnglesUnits=deg  RotationMatrix=[1 0 0; 0 1 0; 0 0 1]  Quaternion=[1 0 0 0]
  Universal SpringL Body : sm_lib/Joints/Universal Joint  JointMode=Normal  SenseConstraintForce=off  SenseConstraintForceX=off  SenseConstraintForceY=off  SenseConstraintForceZ=off  SenseConstraintTorque=off  SenseConstraintTorqueX=off  SenseConstraintTorqueY=off  SenseConstraintTorqueZ=off  SenseTotalForce=off  SenseTotalForceX=off  SenseTotalForceY=off  SenseTotalForceZ=off  SenseTotalTorque=off  SenseTotalTorqueX=off  SenseTotalTorqueY=off  SenseTotalTorqueZ=off  CompositeWrenchDir=FollowerOnBase  CompositeWrenchFrame=BaseFrame  RxEquilibriumPosition=0  RxEquilibriumPositionUnits=deg  RxSpringStiffness=0  RxSpringStiffnessUnits=N*m/deg  RxDampingCoefficient=0  RxDampingCoefficientUnits=N*m/(deg/s)  RxTorqueActuationMode=NoTorque  RxMotionActuationMode=ComputedMotion  RxSensePosition=off  RxSenseVelocity=off  RxSenseAcceleration=off  RxSenseTorqueForce=off  RxSenseLowerLimitTorqueForce=off  RxSenseUpperLimitTorqueForce=off  RxLowerLimitSpecify=off  RxLowerLimitBound=-90  RxLowerLimitBoundUnits=deg  RxLowerLimitStiffness=1e4  RxLowerLimitStiffnessUnits=N*m/deg  RxLowerLimitDamping=10  RxLowerLimitDampingUnits=N*m/(deg/s)  RxLowerLimitTransitionRegionWidth=0.1  RxLowerLimitTransitionRegionWidthUnits=deg  RxUpperLimitSpecify=off  RxUpperLimitBound=90  RxUpperLimitBoundUnits=deg  RxUpperLimitStiffness=1e4  RxUpperLimitStiffnessUnits=N*m/deg  RxUpperLimitDamping=10  RxUpperLimitDampingUnits=N*m/(deg/s)  RxUpperLimitTransitionRegionWidth=0.1  RxUpperLimitTransitionRegionWidthUnits=deg  RxPositionTargetSpecify=off  RxPositionTargetPriority=High  RxPositionTargetValue=0  RxPositionTargetValueUnits=deg  RxVelocityTargetSpecify=off  RxVelocityTargetPriority=High  RxVelocityTargetValue=0  RxVelocityTargetValueUnits=deg/s  RyEquilibriumPosition=0  RyEquilibriumPositionUnits=deg  RySpringStiffness=0  RySpringStiffnessUnits=N*m/deg  RyDampingCoefficient=0  RyDampingCoefficientUnits=N*m/(deg/s)  RyTorqueActuationMode=NoTorque  RyMotionActuationMode=ComputedMotion  RySensePosition=off  RySenseVelocity=off  RySenseAcceleration=off  RySenseTorqueForce=off  RySenseLowerLimitTorqueForce=off  RySenseUpperLimitTorqueForce=off  RyLowerLimitSpecify=off  RyLowerLimitBound=-90  RyLowerLimitBoundUnits=deg  RyLowerLimitStiffness=1e4  RyLowerLimitStiffnessUnits=N*m/deg  RyLowerLimitDamping=10  RyLowerLimitDampingUnits=N*m/(deg/s)  RyLowerLimitTransitionRegionWidth=0.1  RyLowerLimitTransitionRegionWidthUnits=deg  RyUpperLimitSpecify=off  RyUpperLimitBound=90  RyUpperLimitBoundUnits=deg  RyUpperLimitStiffness=1e4  RyUpperLimitStiffnessUnits=N*m/deg  RyUpperLimitDamping=10  RyUpperLimitDampingUnits=N*m/(deg/s)  RyUpperLimitTransitionRegionWidth=0.1  RyUpperLimitTransitionRegionWidthUnits=deg  RyPositionTargetSpecify=off  RyPositionTargetPriority=High  RyPositionTargetValue=0  RyPositionTargetValueUnits=deg  RyVelocityTargetSpecify=off  RyVelocityTargetPriority=High  RyVelocityTargetValue=0  RyVelocityTargetValueUnits=deg/s
  Universal SpringR Body : sm_lib/Joints/Universal Joint  JointMode=Normal  SenseConstraintForce=off  SenseConstraintForceX=off  SenseConstraintForceY=off  SenseConstraintForceZ=off  SenseConstraintTorque=off  SenseConstraintTorqueX=off  SenseConstraintTorqueY=off  SenseConstraintTorqueZ=off  SenseTotalForce=off  SenseTotalForceX=off  SenseTotalForceY=off  SenseTotalForceZ=off  SenseTotalTorque=off  SenseTotalTorqueX=off  SenseTotalTorqueY=off  SenseTotalTorqueZ=off  CompositeWrenchDir=FollowerOnBase  CompositeWrenchFrame=BaseFrame  RxEquilibriumPosition=0  RxEquilibriumPositionUnits=deg  RxSpringStiffness=0  RxSpringStiffnessUnits=N*m/deg  RxDampingCoefficient=0  RxDampingCoefficientUnits=N*m/(deg/s)  RxTorqueActuationMode=NoTorque  RxMotionActuationMode=ComputedMotion  RxSensePosition=off  RxSenseVelocity=off  RxSenseAcceleration=off  RxSenseTorqueForce=off  RxSenseLowerLimitTorqueForce=off  RxSenseUpperLimitTorqueForce=off  RxLowerLimitSpecify=off  RxLowerLimitBound=-90  RxLowerLimitBoundUnits=deg  RxLowerLimitStiffness=1e4  RxLowerLimitStiffnessUnits=N*m/deg  RxLowerLimitDamping=10  RxLowerLimitDampingUnits=N*m/(deg/s)  RxLowerLimitTransitionRegionWidth=0.1  RxLowerLimitTransitionRegionWidthUnits=deg  RxUpperLimitSpecify=off  RxUpperLimitBound=90  RxUpperLimitBoundUnits=deg  RxUpperLimitStiffness=1e4  RxUpperLimitStiffnessUnits=N*m/deg  RxUpperLimitDamping=10  RxUpperLimitDampingUnits=N*m/(deg/s)  RxUpperLimitTransitionRegionWidth=0.1  RxUpperLimitTransitionRegionWidthUnits=deg  RxPositionTargetSpecify=off  RxPositionTargetPriority=High  RxPositionTargetValue=0  RxPositionTargetValueUnits=deg  RxVelocityTargetSpecify=off  RxVelocityTargetPriority=High  RxVelocityTargetValue=0  RxVelocityTargetValueUnits=deg/s  RyEquilibriumPosition=0  RyEquilibriumPositionUnits=deg  RySpringStiffness=0  RySpringStiffnessUnits=N*m/deg  RyDampingCoefficient=0  RyDampingCoefficientUnits=N*m/(deg/s)  RyTorqueActuationMode=NoTorque  RyMotionActuationMode=ComputedMotion  RySensePosition=off  RySenseVelocity=off  RySenseAcceleration=off  RySenseTorqueForce=off  RySenseLowerLimitTorqueForce=off  RySenseUpperLimitTorqueForce=off  RyLowerLimitSpecify=off  RyLowerLimitBound=-90  RyLowerLimitBoundUnits=deg  RyLowerLimitStiffness=1e4  RyLowerLimitStiffnessUnits=N*m/deg  RyLowerLimitDamping=10  RyLowerLimitDampingUnits=N*m/(deg/s)  RyLowerLimitTransitionRegionWidth=0.1  RyLowerLimitTransitionRegionWidthUnits=deg  RyUpperLimitSpecify=off  RyUpperLimitBound=90  RyUpperLimitBoundUnits=deg  RyUpperLimitStiffness=1e4  RyUpperLimitStiffnessUnits=N*m/deg  RyUpperLimitDamping=10  RyUpperLimitDampingUnits=N*m/(deg/s)  RyUpperLimitTransitionRegionWidth=0.1  RyUpperLimitTransitionRegionWidthUnits=deg  RyPositionTargetSpecify=off  RyPositionTargetPriority=High  RyPositionTargetValue=0  RyPositionTargetValueUnits=deg  RyVelocityTargetSpecify=off  RyVelocityTargetPriority=High  RyVelocityTargetValue=0  RyVelocityTargetValueUnits=deg/s
  Wheel Meas Left : Suspension_Utilities/Wheel Measurements  popup_leftRight=Left
  Wheel Meas Right : Suspension_Utilities/Wheel Measurements  popup_leftRight=Right
  Ref : PMIOPort  Side=Right
  WCL : PMIOPort  Port=2  Side=Left
  WCR : PMIOPort  Port=3  Side=Right
  AxleL : PMIOPort  Port=4  Side=Left
  AxleR : PMIOPort  Port=5  Side=Right
  SprL : PMIOPort  Port=6  Side=Left
  DmpL : PMIOPort  Port=7  Side=Left
  SprR : PMIOPort  Port=8  Side=Right
  DmpR : PMIOPort  Port=9  Side=Right
  Out Bus Element1 : Outport  VectorParamsAs1DForOutWhenUnconnected=off  PortName=OutBus  Element=DamperL
  Out Bus Element2 : Outport  VectorParamsAs1DForOutWhenUnconnected=off  PortName=OutBus  Element=DamperR
  Out Bus Element3 : Outport  VectorParamsAs1DForOutWhenUnconnected=off  PortName=OutBus  Element=Bumpstop
  Out Bus Element4 : Outport  VectorParamsAs1DForOutWhenUnconnected=off  PortName=OutBus  Element=SpringR
  Out Bus Element5 : Outport  VectorParamsAs1DForOutWhenUnconnected=off  PortName=OutBus  Element=SpringL
  Out Bus Element6 : Outport  VectorParamsAs1DForOutWhenUnconnected=off  PortName=OutBus  Element=Steer
  Out Bus Element7 : Outport  VectorParamsAs1DForOutWhenUnconnected=off  PortName=OutBus  Element=WhlL
  Out Bus Element8 : Outport  VectorParamsAs1DForOutWhenUnconnected=off  PortName=OutBus  Element=WhlR
  Out Bus Element9 : Outport  VectorParamsAs1DForOutWhenUnconnected=off  PortName=OutBus  Element=DprBR
  Out Bus Element10 : Outport  VectorParamsAs1DForOutWhenUnconnected=off  PortName=OutBus  Element=DprAR
  Out Bus Element11 : Outport  VectorParamsAs1DForOutWhenUnconnected=off  PortName=OutBus  Element=TABR
  Out Bus Element12 : Outport  VectorParamsAs1DForOutWhenUnconnected=off  PortName=OutBus  Element=PanB
  Out Bus Element13 : Outport  VectorParamsAs1DForOutWhenUnconnected=off  PortName=OutBus  Element=PanA
  Out Bus Element14 : Outport  VectorParamsAs1DForOutWhenUnconnected=off  PortName=OutBus  Element=TABL
  Out Bus Element15 : Outport  VectorParamsAs1DForOutWhenUnconnected=off  PortName=OutBus  Element=DprBL
  Out Bus Element16 : Outport  VectorParamsAs1DForOutWhenUnconnected=off  PortName=OutBus  Element=DprAL
  wires:
  Bus Element In1/1 -> Terminator1/1
  Bus Element In/1 -> Terminator/1
  DamperR/1 -> Out Bus Element2/1
  Wheel Meas Right/1 -> Out Bus Element8/1
  Wheel Meas Left/1 -> Out Bus Element7/1
  DamperL/1 -> Out Bus Element1/1
  Bumpstop/1 -> Out Bus Element3/1
  SpringR/1 -> Out Bus Element4/1
  SpringL/1 -> Out Bus Element5/1
  Revolute L/1 -> Terminator3/1
  Revolute R/1 -> Terminator2/1
  Meas/1 -> Out Bus Element6/1
  HP DamperR Body/1 -> Out Bus Element9/1
  HP DamperR Axle/1 -> Out Bus Element10/1
  HP ArmR Gimbal/1 -> Out Bus Element11/1
  HP Pan Body/1 -> Out Bus Element12/1
  HP Pan Axle/1 -> Out Bus Element13/1
  HP ArmL Gimbal/1 -> Out Bus Element14/1
  HP DamperL Body/1 -> Out Bus Element15/1
  HP DamperL Axle/1 -> Out Bus Element16/1
  connections:
  HP DamperL Body/RConn1 -- Hardpoints/RConn1
  Hardpoints/RConn8 -- HP DamperR Body/RConn1
  DmpR/RConn1 -- DamperR/RConn1
  AxleR/RConn1 -- Simscape Bus L/RConn1
  Transform sWheelCtrR/LConn1 -- Wheel Meas Right/LConn2 -- WCR/RConn1 -- HP WC R/RConn1 -- Stub Axle R/LConn1
  AxleL/RConn1 -- Simscape Bus L1/RConn1
  Transform sWheelCtrL/LConn1 -- WCL/RConn1 -- Wheel Meas Left/LConn2 -- Stub Axle L/LConn1 -- HP WC L/RConn1
  Ref/RConn1 -- Connection Label/LConn1 -- Hardpoints/LConn1 -- HP Ref/RConn1
  HP ArmR Gimbal/LConn1 -- Trailing ArmR/RConn1
  HP ArmR Gimbal/RConn1 -- Hardpoints/RConn6
  HP Pan Axle/LConn1 -- Panhard Rod/LConn1
  Panhard Rod/RConn1 -- HP Pan Body/LConn1
  Hardpoints/RConn4 -- HP Pan Body/RConn1
  Axle/RConn4 -- HP Pan Axle/RConn1
  HP DamperL Axle/LConn1 -- Axle/RConn1
  HP DamperR Axle/LConn1 -- Axle/RConn8
  Arm to AxleL/LConn1 -- Trailing ArmL/LConn1
  Arm to AxleL/RConn1 -- Axle/RConn3
  Arm to AxleR/LConn1 -- Trailing ArmR/LConn1
  Arm to AxleR/RConn1 -- Axle/RConn6
  Connection Label1/LConn1 -- Wheel Meas Right/LConn1 -- Wheel Meas Left/LConn1
  HP DamperR Axle/RConn1 -- DamperR/LConn1
  DamperR/RConn2 -- HP DamperR Body/LConn1
  HP DamperL Axle/RConn1 -- DamperL/LConn1
  DamperL/RConn2 -- HP DamperL Body/LConn1
  DamperL/RConn1 -- DmpL/RConn1
  Hardpoints/RConn5 -- Bumpstop/LConn1
  Bumpstop/RConn1 -- Axle/RConn5
  Universal SpringL Body/RConn1 -- SpringL/RConn2
  SpringL/LConn1 -- Spherical SpringL Axle/RConn1
  Hardpoints/RConn2 -- Universal SpringL Body/LConn1
  SprL/RConn1 -- SpringL/RConn1
  Spherical SpringR Axle/RConn1 -- SpringR/LConn1
  Universal SpringR Body/RConn1 -- SpringR/RConn2
  Spherical SpringR Axle/LConn1 -- Axle/RConn7
  Universal SpringR Body/LConn1 -- Hardpoints/RConn7
  SprR/RConn1 -- SpringR/RConn1
  Transform sWheelCtrR/RConn1 -- Simscape Bus L/LConn1 -- Revolute R/LConn2
  Transform sWheelCtrL/RConn1 -- Simscape Bus L1/LConn1 -- Revolute L/LConn2
  Bearing Carrier L/RConn1 -- Simscape Bus L1/LConn2 -- Axle/LConn1 -- Revolute L/RConn1
  Bearing Carrier R/RConn1 -- Simscape Bus L/LConn2 -- Axle/LConn3 -- Revolute R/RConn1
  Simscape Bus L/LConn3 -- Revolute R/LConn1
  Revolute L/LConn1 -- Simscape Bus L1/LConn3
  Simscape Bus L1/LConn4 -- Stub Axle L/RConn1
  Stub Axle R/RConn1 -- Simscape Bus L/LConn4
  Spherical SpringL Axle/LConn1 -- Axle/RConn2
  HP ArmL Gimbal/LConn1 -- Trailing ArmL/RConn1
  Hardpoints/RConn3 -- HP ArmL Gimbal/RConn1

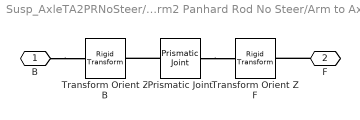
== system Susp_AxleTA2PRNoSteer/Axle Arm2 Panhard Rod No Steer/Arm to AxleL ==
  Prismatic Joint : sm_lib/Joints/Prismatic Joint  JointMode=Normal  SenseConstraintForce=off  SenseConstraintForceX=off  SenseConstraintForceY=off  SenseConstraintForceZ=off  SenseConstraintTorque=off  SenseConstraintTorqueX=off  SenseConstraintTorqueY=off  SenseConstraintTorqueZ=off  SenseTotalForce=off  SenseTotalForceX=off  SenseTotalForceY=off  SenseTotalForceZ=off  SenseTotalTorque=off  SenseTotalTorqueX=off  SenseTotalTorqueY=off  SenseTotalTorqueZ=off  CompositeWrenchDir=FollowerOnBase  CompositeWrenchFrame=BaseFrame  EquilibriumPosition=0  EquilibriumPositionUnits=m  SpringStiffness=0  SpringStiffnessUnits=N/m  DampingCoefficient=0  DampingCoefficientUnits=N/(m/s)  TorqueActuationMode=NoTorque  MotionActuationMode=ComputedMotion  SensePosition=off  SenseVelocity=off  SenseAcceleration=off  SenseTorqueForce=off  SenseLowerLimitTorqueForce=off  SenseUpperLimitTorqueForce=off  LowerLimitSpecify=off  LowerLimitBound=-1  LowerLimitBoundUnits=m  LowerLimitStiffness=1e6  LowerLimitStiffnessUnits=N/m  LowerLimitDamping=1e3  LowerLimitDampingUnits=N/(m/s)  LowerLimitTransitionRegionWidth=1e-4  LowerLimitTransitionRegionWidthUnits=m  UpperLimitSpecify=off  UpperLimitBound=1  UpperLimitBoundUnits=m  UpperLimitStiffness=1e6  UpperLimitStiffnessUnits=N/m  UpperLimitDamping=1e3  UpperLimitDampingUnits=N/(m/s)  UpperLimitTransitionRegionWidth=1e-4  UpperLimitTransitionRegionWidthUnits=m  PositionTargetSpecify=off  PositionTargetPriority=High  PositionTargetValue=0  PositionTargetValueUnits=m  VelocityTargetSpecify=off  VelocityTargetPriority=High  VelocityTargetValue=0  VelocityTargetValueUnits=m/s
  Transform Orient Z B : sm_lib/Frames and Transforms/Rigid Transform  TranslationMethod=None  TranslationStandardOffset=0  TranslationStandardOffsetUnits=m  TranslationStandardAxis=+Z  TranslationCartesianOffset=[0 0 0]  TranslationCartesianOffsetUnits=m  TranslationROffset=0  TranslationROffsetUnits=m  TranslationZOffset=0  TranslationZOffsetUnits=m  TranslationThetaOffset=0  TranslationThetaOffsetUnits=deg  RotationMethod=StandardAxis  RotationAngleUnits=deg  RotationStandardAxis=+X  RotationAngle=90  RotationArbitraryAxis=[0 0 1]  FollAlignAxisA=+X  BaseAlignAxisA=+Y  FollAlignAxisB=+Y  BaseAlignAxisB=+Z  RotationSequenceAxes=FollowerAxes  RotationSequence=XYX  RotationSequenceAngles=[0 0 0]  RotationSequenceAnglesUnits=deg  RotationMatrix=[1 0 0;0 1 0;0 0 1]  Quaternion=[1 0 0 0]
  Transform Orient Z F : sm_lib/Frames and Transforms/Rigid Transform  TranslationMethod=None  TranslationStandardOffset=0  TranslationStandardOffsetUnits=m  TranslationStandardAxis=+Z  TranslationCartesianOffset=[0 0 0]  TranslationCartesianOffsetUnits=m  TranslationROffset=0  TranslationROffsetUnits=m  TranslationZOffset=0  TranslationZOffsetUnits=m  TranslationThetaOffset=0  TranslationThetaOffsetUnits=deg  RotationMethod=StandardAxis  RotationAngleUnits=deg  RotationStandardAxis=+X  RotationAngle=90  RotationArbitraryAxis=[0 0 1]  FollAlignAxisA=+X  BaseAlignAxisA=+Y  FollAlignAxisB=+Y  BaseAlignAxisB=+Z  RotationSequenceAxes=FollowerAxes  RotationSequence=XYX  RotationSequenceAngles=[0 0 0]  RotationSequenceAnglesUnits=deg  RotationMatrix=[1 0 0;0 1 0;0 0 1]  Quaternion=[1 0 0 0]
  B : PMIOPort  Side=Left
  F : PMIOPort  Port=2  Side=Right
  connections:
  B/RConn1 -- Transform Orient Z B/LConn1
  Prismatic Joint/LConn1 -- Transform Orient Z B/RConn1
  Prismatic Joint/RConn1 -- Transform Orient Z F/RConn1
  F/RConn1 -- Transform Orient Z F/LConn1

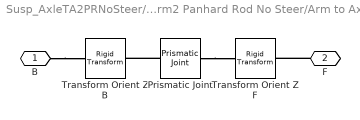
== system Susp_AxleTA2PRNoSteer/Axle Arm2 Panhard Rod No Steer/Arm to AxleR ==
  Prismatic Joint : sm_lib/Joints/Prismatic Joint  JointMode=Normal  SenseConstraintForce=off  SenseConstraintForceX=off  SenseConstraintForceY=off  SenseConstraintForceZ=off  SenseConstraintTorque=off  SenseConstraintTorqueX=off  SenseConstraintTorqueY=off  SenseConstraintTorqueZ=off  SenseTotalForce=off  SenseTotalForceX=off  SenseTotalForceY=off  SenseTotalForceZ=off  SenseTotalTorque=off  SenseTotalTorqueX=off  SenseTotalTorqueY=off  SenseTotalTorqueZ=off  CompositeWrenchDir=FollowerOnBase  CompositeWrenchFrame=BaseFrame  EquilibriumPosition=0  EquilibriumPositionUnits=m  SpringStiffness=0  SpringStiffnessUnits=N/m  DampingCoefficient=0  DampingCoefficientUnits=N/(m/s)  TorqueActuationMode=NoTorque  MotionActuationMode=ComputedMotion  SensePosition=off  SenseVelocity=off  SenseAcceleration=off  SenseTorqueForce=off  SenseLowerLimitTorqueForce=off  SenseUpperLimitTorqueForce=off  LowerLimitSpecify=off  LowerLimitBound=-1  LowerLimitBoundUnits=m  LowerLimitStiffness=1e6  LowerLimitStiffnessUnits=N/m  LowerLimitDamping=1e3  LowerLimitDampingUnits=N/(m/s)  LowerLimitTransitionRegionWidth=1e-4  LowerLimitTransitionRegionWidthUnits=m  UpperLimitSpecify=off  UpperLimitBound=1  UpperLimitBoundUnits=m  UpperLimitStiffness=1e6  UpperLimitStiffnessUnits=N/m  UpperLimitDamping=1e3  UpperLimitDampingUnits=N/(m/s)  UpperLimitTransitionRegionWidth=1e-4  UpperLimitTransitionRegionWidthUnits=m  PositionTargetSpecify=off  PositionTargetPriority=High  PositionTargetValue=0  PositionTargetValueUnits=m  VelocityTargetSpecify=off  VelocityTargetPriority=High  VelocityTargetValue=0  VelocityTargetValueUnits=m/s
  Transform Orient Z B : sm_lib/Frames and Transforms/Rigid Transform  TranslationMethod=None  TranslationStandardOffset=0  TranslationStandardOffsetUnits=m  TranslationStandardAxis=+Z  TranslationCartesianOffset=[0 0 0]  TranslationCartesianOffsetUnits=m  TranslationROffset=0  TranslationROffsetUnits=m  TranslationZOffset=0  TranslationZOffsetUnits=m  TranslationThetaOffset=0  TranslationThetaOffsetUnits=deg  RotationMethod=StandardAxis  RotationAngleUnits=deg  RotationStandardAxis=+X  RotationAngle=90  RotationArbitraryAxis=[0 0 1]  FollAlignAxisA=+X  BaseAlignAxisA=+Y  FollAlignAxisB=+Y  BaseAlignAxisB=+Z  RotationSequenceAxes=FollowerAxes  RotationSequence=XYX  RotationSequenceAngles=[0 0 0]  RotationSequenceAnglesUnits=deg  RotationMatrix=[1 0 0;0 1 0;0 0 1]  Quaternion=[1 0 0 0]
  Transform Orient Z F : sm_lib/Frames and Transforms/Rigid Transform  TranslationMethod=None  TranslationStandardOffset=0  TranslationStandardOffsetUnits=m  TranslationStandardAxis=+Z  TranslationCartesianOffset=[0 0 0]  TranslationCartesianOffsetUnits=m  TranslationROffset=0  TranslationROffsetUnits=m  TranslationZOffset=0  TranslationZOffsetUnits=m  TranslationThetaOffset=0  TranslationThetaOffsetUnits=deg  RotationMethod=StandardAxis  RotationAngleUnits=deg  RotationStandardAxis=+X  RotationAngle=90  RotationArbitraryAxis=[0 0 1]  FollAlignAxisA=+X  BaseAlignAxisA=+Y  FollAlignAxisB=+Y  BaseAlignAxisB=+Z  RotationSequenceAxes=FollowerAxes  RotationSequence=XYX  RotationSequenceAngles=[0 0 0]  RotationSequenceAnglesUnits=deg  RotationMatrix=[1 0 0;0 1 0;0 0 1]  Quaternion=[1 0 0 0]
  B : PMIOPort  Side=Left
  F : PMIOPort  Port=2  Side=Right
  connections:
  F/RConn1 -- Transform Orient Z F/LConn1
  Prismatic Joint/RConn1 -- Transform Orient Z F/RConn1
  Prismatic Joint/LConn1 -- Transform Orient Z B/RConn1
  B/RConn1 -- Transform Orient Z B/LConn1
